simulink model "px4_controllers_IARTF"  (R2018a)
settings: Solver=ode4  StartTime=0.0  StopTime=sim_time  FixedStep=1/sim_freq  MaxStep=0.0025  MinStep=0.0005  RelTol=1e-3
values from neighbouring files (symbols this model uses):
  C_D = [0.025; 0.025; 0.025]    [quad_parameters_IARTF.m]    (also in quad_parameters_SLADe.m = [0.5; 0.5; 0.5])
  d = 0.1275    [quad_parameters_IARTF.m]    (also in quad_parameters_SLADe.m = 0.465)
  d_step_time = 0    [init_sim.m]
  d_step_val = 0    [init_sim.m]
  e_step_time = 0    [init_sim.m]
  e_step_val = 0    [init_sim.m]
  g = 9.80665    [init_sim.m]
  K_d_D = 0    [controller_gains_IARTF.m]
  K_d_I = 0    [controller_gains_IARTF.m]
  K_d_P = 1.5    [controller_gains_IARTF.m]
  K_e_D = 0    [controller_gains_IARTF.m]
  K_e_I = 0    [controller_gains_IARTF.m]
  K_e_P = 1.5    [controller_gains_IARTF.m]
  K_n_D = 0    [controller_gains_IARTF.m]
  K_n_I = 0    [controller_gains_IARTF.m]
  K_n_P = 1.5    [controller_gains_IARTF.m]
  K_p_D = 0.0135    [controller_gains_IARTF.m]
  K_p_I = 0.789    [controller_gains_IARTF.m]
  K_p_P = 1.466    [controller_gains_IARTF.m]
  K_phi_D = 0    [controller_gains_IARTF.m]
  K_phi_I = 0    [controller_gains_IARTF.m]
  K_phi_P = 8    [controller_gains_IARTF.m]
  K_psi_D = 0    [controller_gains_IARTF.m]
  K_psi_I = 0    [controller_gains_IARTF.m]
  K_psi_P = 4    [controller_gains_IARTF.m]
  K_q_D = 0.0135    [controller_gains_IARTF.m]
  K_q_I = 0.789    [controller_gains_IARTF.m]
  K_q_P = 1.466    [controller_gains_IARTF.m]
  K_r_D = 0    [controller_gains_IARTF.m]
  K_r_I = 0.564    [controller_gains_IARTF.m]
  K_r_P = 1.354    [controller_gains_IARTF.m]
  K_theta_D = 0    [controller_gains_IARTF.m]
  K_theta_I = 0    [controller_gains_IARTF.m]
  K_theta_P = 8    [controller_gains_IARTF.m]
  K_u_D = 0.1128    [controller_gains_IARTF.m]
  K_u_I = 0.2256    [controller_gains_IARTF.m]
  K_u_P = 1.6922    [controller_gains_IARTF.m]
  K_v_D = 0.1128    [controller_gains_IARTF.m]
  K_v_I = 0.2256    [controller_gains_IARTF.m]
  K_v_P = 1.6922    [controller_gains_IARTF.m]
  K_w_D = 0    [controller_gains_IARTF.m]
  K_w_I = 0.15    [controller_gains_IARTF.m]
  K_w_P = 0.8    [controller_gains_IARTF.m]
  m = 1.15    [quad_parameters_IARTF.m]    (also in quad_parameters_SLADe.m = 15)
  n_step_time = 0    [init_sim.m]
  n_step_val = 0    [init_sim.m]
  pitch_rate_step_time = 0    [init_sim.m]
  pitch_rate_step_val = 0    [init_sim.m]
  pitch_step_time = 0    [init_sim.m]
  pitch_step_val = 0    [init_sim.m]
  r_D = 0.115*0.375    (= 0.043125)    [quad_parameters_IARTF.m]    (also in quad_parameters_SLADe.m = 0.18)
  R_LD = 10    [init_sim.m]
  rho = 1.225    [init_sim.m]
  roll_rate_step_time = 0    [init_sim.m]
  roll_rate_step_val = 0    [init_sim.m]
  roll_step_time = 0    [init_sim.m]
  roll_step_val = 0    [init_sim.m]
  vx_step_time = 0    [init_sim.m]
  vx_step_val = 0    [init_sim.m]
  vy_step_time = 0    [init_sim.m]
  vy_step_val = 0    [init_sim.m]
  vz_step_time = 0    [init_sim.m]
  vz_step_val = 0    [init_sim.m]
  yaw_rate_step_time = 0    [init_sim.m]
  yaw_rate_step_val = 0    [init_sim.m]
  yaw_step_time = 0    [init_sim.m]
  yaw_step_val = 0    [init_sim.m]
undefined symbols (not defined in the file or in its folder): A_D, Eul_init, I_b, NED_init, PQR_init, tau, UVW_init
libraries: peGeneralControl x1
settings Model: Creator=Martin  LastModifiedBy=jjr

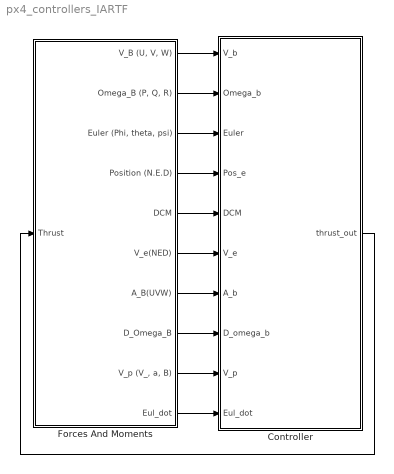
== system px4_controllers_IARTF ==
  Controller : Subsystem
  Forces And Moments : Subsystem
  wires:
  Forces And Moments/1("V_B (U, V, W)") -> Controller/1(V_b)
  Forces And Moments/2("Omega_B (P, Q, R)") -> Controller/2(Omega_b)
  Forces And Moments/3("Euler (Phi, theta, psi)") -> Controller/3(Euler)
  Forces And Moments/4(Position (N.E.D)) -> Controller/4(Pos_e)
  Forces And Moments/5(DCM) -> Controller/5(DCM)
  Forces And Moments/6(V_e(NED)) -> Controller/6(V_e)
  Forces And Moments/7(A_B(UVW)) -> Controller/7(A_b)
  Forces And Moments/8(D_Omega_B) -> Controller/8(D_omega_b)
  Forces And Moments/9("V_p (V_, a, B)") -> Controller/9(V_p)
  Forces And Moments/10(Eul_dot) -> Controller/10(Eul_dot)
  Controller/1(thrust_out) -> Forces And Moments/1(Thrust)

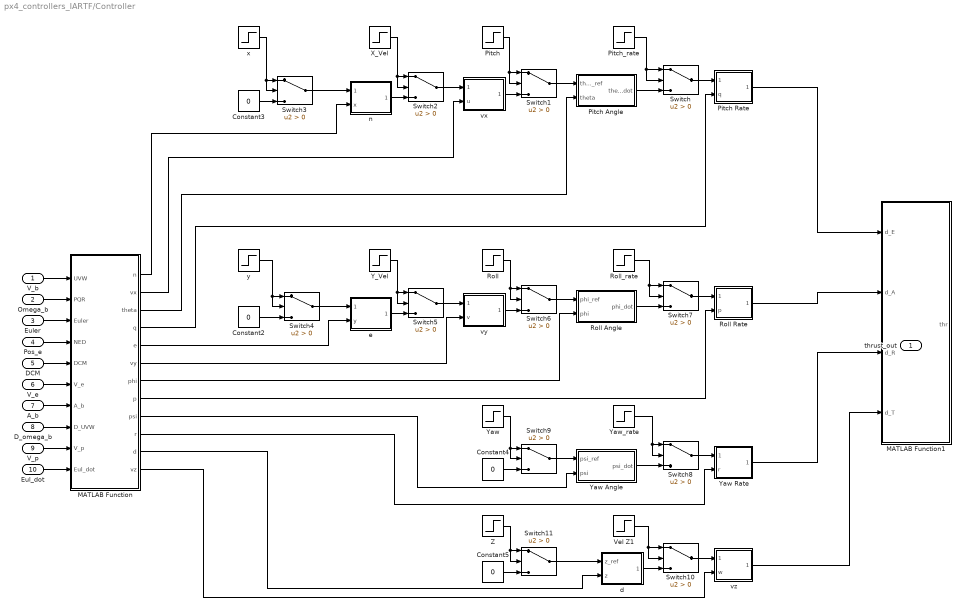
== system px4_controllers_IARTF/Controller ==
  V_b : Inport
  Omega_b : Inport  Port=2
  Euler : Inport  Port=3
  Pos_e : Inport  Port=4
  DCM : Inport  Port=5
  V_e : Inport  Port=6
  A_b : Inport  Port=7
  D_omega_b : Inport  Port=8
  V_p : Inport  Port=9
  Eul_dot : Inport  Port=10
  Constant{2..5} (4 alike) : Constant  Value=0
  MATLAB Function : MATLAB Function  TreatAsAtomicUnit=on
  MATLAB Function1 : MATLAB Function  TreatAsAtomicUnit=on
  Pitch : Step  Time=pitch_step_time  After=pitch_step_val  SampleTime=0
  Pitch Angle : Subsystem
  Pitch Rate : Subsystem
  Pitch_rate : Step  Time=pitch_rate_step_time  After=pitch_rate_step_val  SampleTime=0
  Roll : Step  Time=roll_step_time  After=roll_step_val  SampleTime=0
  Roll Angle : Subsystem
  Roll Rate : Subsystem
  Roll_rate : Step  Time=roll_rate_step_time  After=roll_rate_step_val  SampleTime=0
  Switch{,1..11} (12 alike) : Switch  Criteria=u2 > Threshold
  Vel Z1 : Step  Time=vz_step_time  After=vz_step_val  SampleTime=0
  X_Vel : Step  Time=vx_step_time  After=vx_step_val  SampleTime=0
  Y_Vel : Step  Time=vy_step_time  After=vy_step_val  SampleTime=0
  Yaw : Step  Time=yaw_step_time  After=yaw_step_val  SampleTime=0
  Yaw Angle : Subsystem
  Yaw Rate : Subsystem
  Yaw_rate : Step  Time=yaw_rate_step_time  After=yaw_rate_step_val  SampleTime=0
  Z : Step  Time=d_step_time  After=d_step_val  SampleTime=0
  d : Subsystem
  e : Subsystem
  n : Subsystem
  vx : Subsystem
  vy : Subsystem
  vz : Subsystem
  x : Step  Time=n_step_time  After=n_step_val  SampleTime=0
  y : Step  Time=e_step_time  After=e_step_val  SampleTime=0
  thrust_out : Outport
  wires:
  Switch2/1 -> vx/1(u_ref)
  Pitch/1 -> Switch1/2, Switch1/1
  Pitch_rate/1 -> Switch/2, Switch/1
  Pitch Angle/1(theta_dot) -> Switch/3
  vx/1(u_dot) -> Switch1/3
  d/1(d_dot) -> Switch10/3
  Switch11/1 -> d/1(z_ref)
  Yaw/1 -> Switch9/2, Switch9/1
  e/1(y_dot) -> Switch5/3
  Z/1 -> Switch11/2, Switch11/1
  Constant2/1 -> Switch4/3
  Yaw Angle/1(psi_dot) -> Switch8/3
  Switch3/1 -> n/1(X_ref)
  n/1(x_dot) -> Switch2/3
  Roll Rate/1(p_dot) -> MATLAB Function1/2(d_A)
  Yaw_rate/1 -> Switch8/2, Switch8/1
  X_Vel/1 -> Switch2/2, Switch2/1
  vy/1(v_dot) -> Switch6/3
  Switch4/1 -> e/1(Y_ref)
  Constant4/1 -> Switch9/3
  Vel Z1/1 -> Switch10/2, Switch10/1
  Pitch Rate/1(q_dot) -> MATLAB Function1/1(d_E)
  Constant3/1 -> Switch3/3
  Switch5/1 -> vy/1(v_ref)
  Switch9/1 -> Yaw Angle/1(psi_ref)
  Y_Vel/1 -> Switch5/1, Switch5/2
  y/1 -> Switch4/2, Switch4/1
  Switch6/1 -> Roll Angle/1(phi_ref)
  Switch7/1 -> Roll Rate/1(p_ref)
  Switch10/1 -> vz/1(w_ref)
  x/1 -> Switch3/2, Switch3/1
  Switch8/1 -> Yaw Rate/1(r_ref)
  Switch1/1 -> Pitch Angle/1(theta_ref)
  Roll Angle/1(phi_dot) -> Switch7/3
  Roll/1 -> Switch6/1, Switch6/2
  Roll_rate/1 -> Switch7/2, Switch7/1
  Constant5/1 -> Switch11/3
  Yaw Rate/1(r_dot) -> MATLAB Function1/3(d_R)
  Switch/1 -> Pitch Rate/1(q_ref)
  Eul_dot/1 -> MATLAB Function/10(Eul_dot)
  V_b/1 -> MATLAB Function/1(UVW)
  Omega_b/1 -> MATLAB Function/2(PQR)
  Euler/1 -> MATLAB Function/3(Euler)
  Pos_e/1 -> MATLAB Function/4(NED)
  DCM/1 -> MATLAB Function/5(DCM)
  V_e/1 -> MATLAB Function/6(V_e)
  A_b/1 -> MATLAB Function/7(A_b)
  D_omega_b/1 -> MATLAB Function/8(D_UVW)
  V_p/1 -> MATLAB Function/9(V_p)
  MATLAB Function/1(n) -> n/2(x)
  MATLAB Function/2(vx) -> vx/2(u)
  MATLAB Function/3(theta) -> Pitch Angle/2(theta)
  MATLAB Function/4(q) -> Pitch Rate/2(q)
  MATLAB Function/5(e) -> e/2(y)
  MATLAB Function/6(vy) -> vy/2(v)
  MATLAB Function/7(phi) -> Roll Angle/2(phi)
  MATLAB Function/8(p) -> Roll Rate/2(p)
  MATLAB Function/9(psi) -> Yaw Angle/2(psi)
  MATLAB Function/10(r) -> Yaw Rate/2(r)
  vz/1(w_dot) -> MATLAB Function1/4(d_T)
  MATLAB Function/11(d) -> d/2(z)
  MATLAB Function/12(vz) -> vz/2(w)

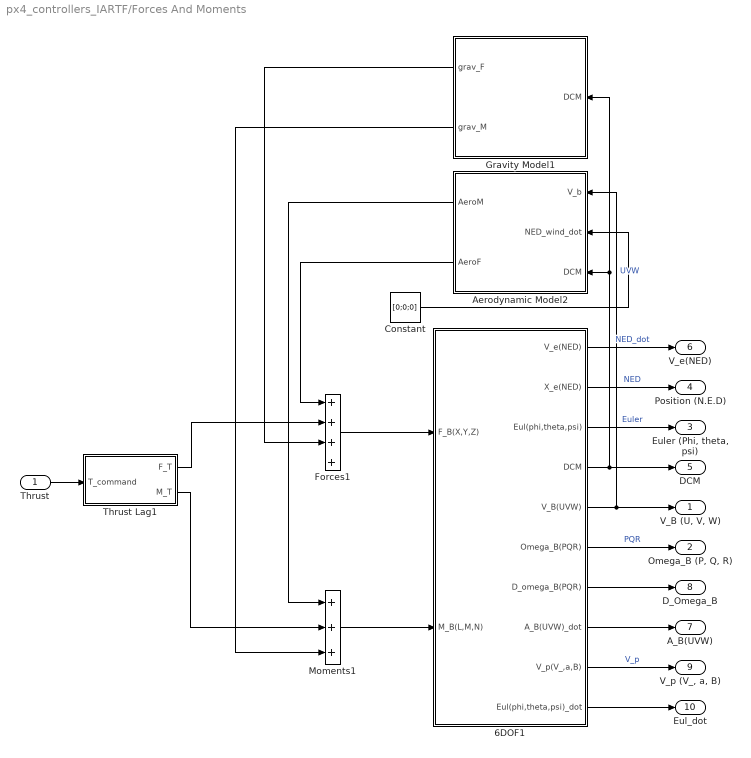
== system px4_controllers_IARTF/Forces And Moments ==
  Thrust : Inport
  6DOF1 : Subsystem
  Aerodynamic Model2 : MATLAB Function  TreatAsAtomicUnit=on
  Constant : Constant  Value=[0;0;0]
  Forces1 : Sum  Inputs=++++  RndMeth=Nearest
  Gravity Model1 : MATLAB Function  TreatAsAtomicUnit=on
  Moments1 : Sum  Inputs=+++  RndMeth=Nearest
  Thrust Lag1 : Subsystem
  "V_B (U, V, W)" : Outport
  "Omega_B (P, Q, R)" : Outport  Port=2
  "Euler (Phi, theta, psi)" : Outport  Port=3
  Position (N.E.D) : Outport  Port=4
  DCM : Outport  Port=5
  V_e(NED) : Outport  Port=6
  A_B(UVW) : Outport  Port=7
  D_Omega_B : Outport  Port=8
  "V_p (V_, a, B)" : Outport  Port=9
  Eul_dot : Outport  Port=10
  wires:
  Thrust/1 -> Thrust Lag1/1(T_command)
  6DOF1/3(Eul(phi,theta,psi)) -> "Euler (Phi, theta, psi)"/1  "Euler"
  Constant/1 -> Aerodynamic Model2/2(NED_wind_dot)
  Aerodynamic Model2/1(AeroM) -> Moments1/1
  Moments1/1 -> 6DOF1/2(M_B(L,M,N))
  Thrust Lag1/1(F_T) -> Forces1/2
  Gravity Model1/2(grav_M) -> Moments1/3
  Thrust Lag1/2(M_T) -> Moments1/2
  6DOF1/4(DCM) -> Gravity Model1/1(DCM), Aerodynamic Model2/3(DCM), DCM/1
  6DOF1/9(V_p(V_,a,B)) -> "V_p (V_, a, B)"/1  "V_p"
  Forces1/1 -> 6DOF1/1(F_B(X,Y,Z))
  Aerodynamic Model2/2(AeroF) -> Forces1/1
  6DOF1/6(Omega_B(PQR)) -> "Omega_B (P, Q, R)"/1  "PQR"
  6DOF1/10(Eul(phi,theta,psi)_dot) -> Eul_dot/1
  6DOF1/8(A_B(UVW)_dot) -> A_B(UVW)/1
  Gravity Model1/1(grav_F) -> Forces1/3
  6DOF1/5(V_B(UVW)) -> "V_B (U, V, W)"/1, Aerodynamic Model2/1(V_b)  "UVW"
  6DOF1/2(X_e(NED)) -> Position (N.E.D)/1  "NED"
  6DOF1/7(D_omega_B(PQR)) -> D_Omega_B/1
  6DOF1/1(V_e(NED)) -> V_e(NED)/1  "NED_dot"

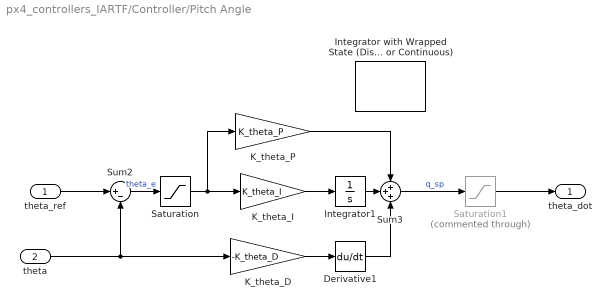
== system px4_controllers_IARTF/Controller/Pitch Angle ==
  theta_ref : Inport
  theta : Inport  Port=2
  Derivative1 : Derivative
  Integrator with Wrapped State (Discrete or Continuous) : peGeneralControl/Integrator with Wrapped State (Discrete or Continuous)  OverrideUsingVariant=Discrete  WrappedStateUpperValue=2*pi  WrappedStateLowerValue=0  x0=0  Ts=-1
  Integrator1 : Integrator
  K_theta_D : Gain  Gain=-K_theta_D
  K_theta_I : Gain  Gain=K_theta_I
  K_theta_P : Gain  Gain=K_theta_P
  Saturation : Saturate  UpperLimit=pi/6  LowerLimit=-pi/6
  Saturation1 : Saturate  Commented=through  UpperLimit=1  LowerLimit=-1
  Sum2 : Sum  Inputs=|+-
  Sum3 : Sum  Inputs=+++
  theta_dot : Outport
  wires:
  Saturation1/1 -> theta_dot/1
  Saturation/1 -> K_theta_P/1, K_theta_I/1
  Derivative1/1 -> Sum3/3
  Integrator1/1 -> Sum3/2
  Sum3/1 -> Saturation1/1  "q_sp"
  K_theta_I/1 -> Integrator1/1
  Sum2/1 -> Saturation/1  "theta_e"
  K_theta_P/1 -> Sum3/1
  K_theta_D/1 -> Derivative1/1
  theta_ref/1 -> Sum2/1
  theta/1 -> K_theta_D/1, Sum2/2

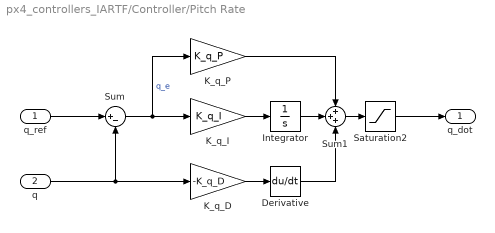
== system px4_controllers_IARTF/Controller/Pitch Rate ==
  q_ref : Inport
  q : Inport  Port=2
  Derivative : Derivative
  Integrator : Integrator
  K_q_D : Gain  Gain=-K_q_D
  K_q_I : Gain  Gain=K_q_I
  "K_q_P " : Gain  Gain=K_q_P
  Saturation2 : Saturate  UpperLimit=1  LowerLimit=-1
  Sum : Sum  Inputs=|+-
  Sum1 : Sum  Inputs=+++
  q_dot : Outport
  wires:
  Integrator/1 -> Sum1/2
  Derivative/1 -> Sum1/3
  "K_q_P "/1 -> Sum1/1
  K_q_D/1 -> Derivative/1
  K_q_I/1 -> Integrator/1
  Sum1/1 -> Saturation2/1
  Sum/1 -> "K_q_P "/1, K_q_I/1  "q_e"
  q_ref/1 -> Sum/1
  Saturation2/1 -> q_dot/1
  q/1 -> K_q_D/1, Sum/2

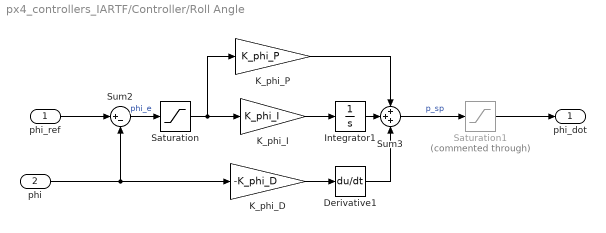
== system px4_controllers_IARTF/Controller/Roll Angle ==
  phi_ref : Inport
  phi : Inport  Port=2
  Derivative1 : Derivative
  Integrator1 : Integrator
  K_phi_D : Gain  Gain=-K_phi_D
  K_phi_I : Gain  Gain=K_phi_I
  K_phi_P : Gain  Gain=K_phi_P
  Saturation : Saturate  UpperLimit=pi/6  LowerLimit=-pi/6
  Saturation1 : Saturate  Commented=through  UpperLimit=1  LowerLimit=-1
  Sum2 : Sum  Inputs=|+-
  Sum3 : Sum  Inputs=+++
  phi_dot : Outport
  wires:
  Saturation1/1 -> phi_dot/1
  Saturation/1 -> K_phi_P/1, K_phi_I/1
  Derivative1/1 -> Sum3/3
  Integrator1/1 -> Sum3/2
  Sum3/1 -> Saturation1/1  "p_sp"
  K_phi_I/1 -> Integrator1/1
  Sum2/1 -> Saturation/1  "phi_e"
  K_phi_P/1 -> Sum3/1
  K_phi_D/1 -> Derivative1/1
  phi_ref/1 -> Sum2/1
  phi/1 -> K_phi_D/1, Sum2/2

== system px4_controllers_IARTF/Controller/Roll Rate ==
  p_ref : Inport
  p : Inport  Port=2
  Derivative : Derivative
  Integrator : Integrator
  K_p_D : Gain  Gain=-K_p_D
  K_p_I : Gain  Gain=K_p_I
  "K_p_P " : Gain  Gain=K_p_P
  Saturation2 : Saturate  UpperLimit=1  LowerLimit=-1
  Sum : Sum  Inputs=|+-
  Sum1 : Sum  Inputs=+++
  p_dot : Outport
  wires:
  Integrator/1 -> Sum1/2
  Derivative/1 -> Sum1/3
  "K_p_P "/1 -> Sum1/1
  K_p_D/1 -> Derivative/1
  K_p_I/1 -> Integrator/1
  Sum1/1 -> Saturation2/1
  Sum/1 -> "K_p_P "/1, K_p_I/1  "p_e"
  p_ref/1 -> Sum/1
  Saturation2/1 -> p_dot/1
  p/1 -> K_p_D/1, Sum/2

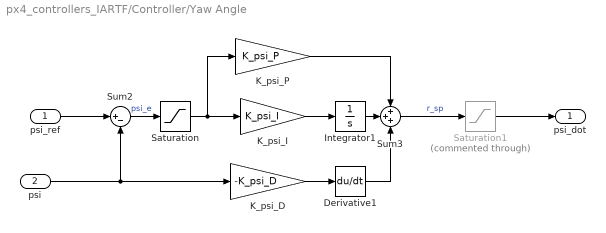
== system px4_controllers_IARTF/Controller/Yaw Angle ==
  psi_ref : Inport
  psi : Inport  Port=2
  Derivative1 : Derivative
  Integrator1 : Integrator
  K_psi_D : Gain  Gain=-K_psi_D
  K_psi_I : Gain  Gain=K_psi_I
  K_psi_P : Gain  Gain=K_psi_P
  Saturation : Saturate  UpperLimit=pi/6  LowerLimit=-pi/6
  Saturation1 : Saturate  Commented=through  UpperLimit=1  LowerLimit=-1
  Sum2 : Sum  Inputs=|+-
  Sum3 : Sum  Inputs=+++
  psi_dot : Outport
  wires:
  Saturation1/1 -> psi_dot/1
  Saturation/1 -> K_psi_P/1, K_psi_I/1
  Derivative1/1 -> Sum3/3
  Integrator1/1 -> Sum3/2
  Sum3/1 -> Saturation1/1  "r_sp"
  K_psi_I/1 -> Integrator1/1
  Sum2/1 -> Saturation/1  "psi_e"
  K_psi_P/1 -> Sum3/1
  K_psi_D/1 -> Derivative1/1
  psi_ref/1 -> Sum2/1
  psi/1 -> K_psi_D/1, Sum2/2

== system px4_controllers_IARTF/Controller/Yaw Rate ==
  r_ref : Inport
  r : Inport  Port=2
  Derivative : Derivative
  Integrator : Integrator
  K_r_D : Gain  Gain=-K_r_D
  K_r_I : Gain  Gain=K_r_I
  "K_r_P " : Gain  Gain=K_r_P
  Saturation2 : Saturate  UpperLimit=1  LowerLimit=-1
  Sum : Sum  Inputs=|+-
  Sum1 : Sum  Inputs=+++
  r_dot : Outport
  wires:
  Integrator/1 -> Sum1/2
  Derivative/1 -> Sum1/3
  "K_r_P "/1 -> Sum1/1
  K_r_D/1 -> Derivative/1
  K_r_I/1 -> Integrator/1
  Sum1/1 -> Saturation2/1
  Sum/1 -> "K_r_P "/1, K_r_I/1  "r_e"
  r_ref/1 -> Sum/1
  Saturation2/1 -> r_dot/1
  r/1 -> K_r_D/1, Sum/2

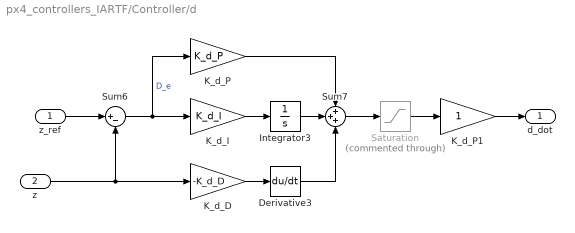
== system px4_controllers_IARTF/Controller/d ==
  z_ref : Inport
  z : Inport  Port=2
  Derivative3 : Derivative
  Integrator3 : Integrator
  K_d_D : Gain  Gain=-K_d_D
  K_d_I : Gain  Gain=K_d_I
  K_d_P : Gain  Gain=K_d_P
  K_d_P1 : Gain
  Saturation : Saturate  Commented=through  UpperLimit=5  LowerLimit=-5
  Sum6 : Sum  Inputs=|+-
  Sum7 : Sum  Inputs=+++
  d_dot : Outport
  wires:
  Saturation/1 -> K_d_P1/1
  K_d_I/1 -> Integrator3/1
  Derivative3/1 -> Sum7/3
  K_d_D/1 -> Derivative3/1
  K_d_P/1 -> Sum7/1
  Integrator3/1 -> Sum7/2
  Sum6/1 -> K_d_P/1, K_d_I/1  "D_e"
  Sum7/1 -> Saturation/1
  z_ref/1 -> Sum6/1
  z/1 -> Sum6/2, K_d_D/1
  K_d_P1/1 -> d_dot/1

== system px4_controllers_IARTF/Controller/e ==
  Y_ref : Inport
  y : Inport  Port=2
  Derivative3 : Derivative
  Integrator3 : Integrator
  K_e_D : Gain  Gain=-K_e_D
  K_e_I : Gain  Gain=K_e_I
  K_e_P : Gain  Gain=K_e_P
  Saturation : Saturate  Commented=through  UpperLimit=5  LowerLimit=-5
  Sum6 : Sum  Inputs=|+-
  Sum7 : Sum  Inputs=+++
  y_dot : Outport
  wires:
  Saturation/1 -> y_dot/1
  K_e_I/1 -> Integrator3/1
  Derivative3/1 -> Sum7/3
  K_e_D/1 -> Derivative3/1
  K_e_P/1 -> Sum7/1
  Integrator3/1 -> Sum7/2
  Sum6/1 -> K_e_P/1, K_e_I/1  "E_e"
  Sum7/1 -> Saturation/1
  Y_ref/1 -> Sum6/1
  y/1 -> K_e_D/1, Sum6/2

== system px4_controllers_IARTF/Controller/n ==
  X_ref : Inport
  x : Inport  Port=2
  Derivative3 : Derivative
  Integrator3 : Integrator
  K_n_D : Gain  Gain=-K_n_D
  K_n_I : Gain  Gain=K_n_I
  K_n_P : Gain  Gain=K_n_P
  Saturation : Saturate  Commented=through  UpperLimit=5  LowerLimit=-5
  Sum6 : Sum  Inputs=|+-
  Sum7 : Sum  Inputs=+++
  x_dot : Outport
  wires:
  Saturation/1 -> x_dot/1
  K_n_I/1 -> Integrator3/1
  Derivative3/1 -> Sum7/3
  K_n_D/1 -> Derivative3/1
  K_n_P/1 -> Sum7/1
  Integrator3/1 -> Sum7/2
  Sum6/1 -> K_n_P/1, K_n_I/1  "N_e"
  Sum7/1 -> Saturation/1
  X_ref/1 -> Sum6/1
  x/1 -> K_n_D/1, Sum6/2

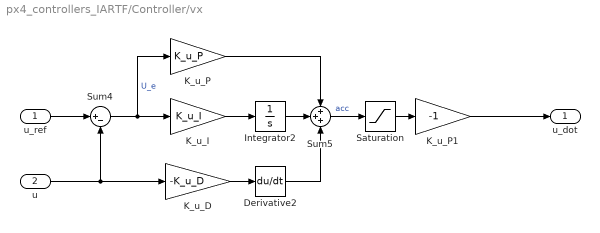
== system px4_controllers_IARTF/Controller/vx ==
  u_ref : Inport
  u : Inport  Port=2
  Derivative2 : Derivative
  Integrator2 : Integrator
  K_u_D : Gain  Gain=-K_u_D
  K_u_I : Gain  Gain=K_u_I
  K_u_P : Gain  Gain=K_u_P
  K_u_P1 : Gain  Gain=-1
  Saturation : Saturate  UpperLimit=5  LowerLimit=-5
  Sum4 : Sum  Inputs=|+-
  Sum5 : Sum  Inputs=+++
  u_dot : Outport
  wires:
  K_u_I/1 -> Integrator2/1
  K_u_P/1 -> Sum5/1
  K_u_D/1 -> Derivative2/1
  Sum4/1 -> K_u_P/1, K_u_I/1  "U_e"
  Sum5/1 -> Saturation/1  "acc"
  Derivative2/1 -> Sum5/3
  Integrator2/1 -> Sum5/2
  u/1 -> K_u_D/1, Sum4/2
  u_ref/1 -> Sum4/1
  Saturation/1 -> K_u_P1/1
  K_u_P1/1 -> u_dot/1

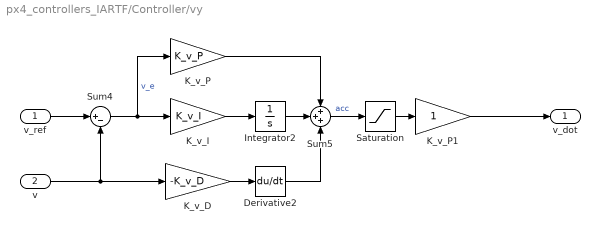
== system px4_controllers_IARTF/Controller/vy ==
  v_ref : Inport
  v : Inport  Port=2
  Derivative2 : Derivative
  Integrator2 : Integrator
  K_v_D : Gain  Gain=-K_v_D
  K_v_I : Gain  Gain=K_v_I
  K_v_P : Gain  Gain=K_v_P
  K_v_P1 : Gain
  Saturation : Saturate  UpperLimit=5  LowerLimit=-5
  Sum4 : Sum  Inputs=|+-
  Sum5 : Sum  Inputs=+++
  v_dot : Outport
  wires:
  K_v_I/1 -> Integrator2/1
  K_v_P/1 -> Sum5/1
  K_v_D/1 -> Derivative2/1
  Sum4/1 -> K_v_P/1, K_v_I/1  "v_e"
  Sum5/1 -> Saturation/1  "acc"
  Derivative2/1 -> Sum5/3
  Integrator2/1 -> Sum5/2
  v/1 -> K_v_D/1, Sum4/2
  v_ref/1 -> Sum4/1
  Saturation/1 -> K_v_P1/1
  K_v_P1/1 -> v_dot/1

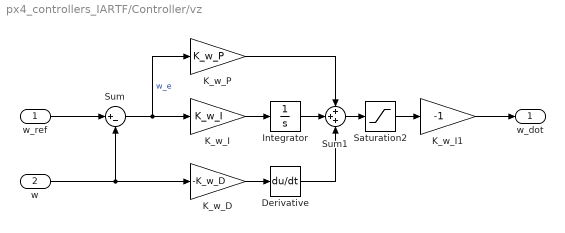
== system px4_controllers_IARTF/Controller/vz ==
  w_ref : Inport
  w : Inport  Port=2
  Derivative : Derivative
  Integrator : Integrator
  K_w_D : Gain  Gain=-K_w_D
  K_w_I : Gain  Gain=K_w_I
  K_w_I1 : Gain  Gain=-1
  "K_w_P " : Gain  Gain=K_w_P
  Saturation2 : Saturate  UpperLimit=1  LowerLimit=-1
  Sum : Sum  Inputs=|+-
  Sum1 : Sum  Inputs=+++
  w_dot : Outport
  wires:
  Integrator/1 -> Sum1/2
  Derivative/1 -> Sum1/3
  "K_w_P "/1 -> Sum1/1
  K_w_D/1 -> Derivative/1
  K_w_I/1 -> Integrator/1
  Sum1/1 -> Saturation2/1
  Sum/1 -> "K_w_P "/1, K_w_I/1  "w_e"
  w_ref/1 -> Sum/1
  Saturation2/1 -> K_w_I1/1
  w/1 -> K_w_D/1, Sum/2
  K_w_I1/1 -> w_dot/1

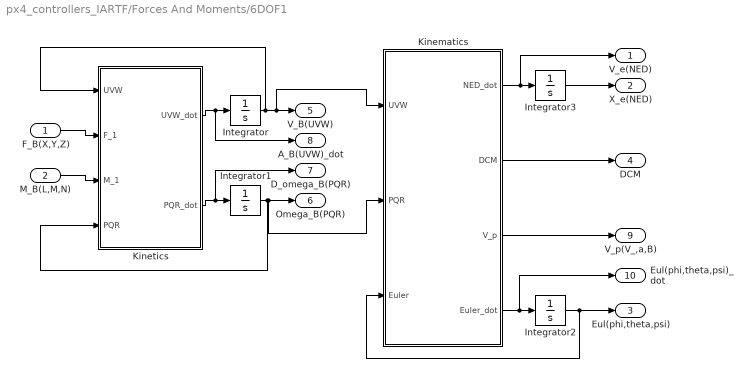
== system px4_controllers_IARTF/Forces And Moments/6DOF1 ==
  F_B(X,Y,Z) : Inport
  M_B(L,M,N) : Inport  Port=2
  Integrator : Integrator  InitialCondition=UVW_init
  Integrator1 : Integrator  InitialCondition=PQR_init
  Integrator2 : Integrator  InitialCondition=Eul_init  WrapState=on  WrappedStateUpperValue=pi.*[1;1;1]  WrappedStateLowerValue=-pi.*[1;1;1]
  Integrator3 : Integrator  InitialCondition=NED_init
  Kinematics : MATLAB Function  TreatAsAtomicUnit=on
  Kinetics : MATLAB Function  TreatAsAtomicUnit=on
  V_e(NED) : Outport
  X_e(NED) : Outport  Port=2
  Eul(phi,theta,psi) : Outport  Port=3
  DCM : Outport  Port=4
  V_B(UVW) : Outport  Port=5
  Omega_B(PQR) : Outport  Port=6
  D_omega_B(PQR) : Outport  Port=7
  A_B(UVW)_dot : Outport  Port=8
  V_p(V_,a,B) : Outport  Port=9
  Eul(phi,theta,psi)_dot : Outport  Port=10
  wires:
  Kinetics/1(UVW_dot) -> A_B(UVW)_dot/1, Integrator/1
  Kinetics/2(PQR_dot) -> D_omega_B(PQR)/1, Integrator1/1
  Integrator1/1 -> Kinetics/4(PQR), Omega_B(PQR)/1, Kinematics/2(PQR)
  Integrator/1 -> Kinetics/1(UVW), Kinematics/1(UVW), V_B(UVW)/1
  M_B(L,M,N)/1 -> Kinetics/3(M_1)
  F_B(X,Y,Z)/1 -> Kinetics/2(F_1)
  Kinematics/4(Euler_dot) -> Eul(phi,theta,psi)_dot/1, Integrator2/1
  Kinematics/3(V_p) -> V_p(V_,a,B)/1
  Kinematics/2(DCM) -> DCM/1
  Kinematics/1(NED_dot) -> V_e(NED)/1, Integrator3/1
  Integrator3/1 -> X_e(NED)/1
  Integrator2/1 -> Kinematics/3(Euler), Eul(phi,theta,psi)/1

== system px4_controllers_IARTF/Forces And Moments/Thrust Lag1 ==
  T_command : Inport
  Integrator : Integrator  InitialCondition=[1;1;1;1].*0
  Trust Model : MATLAB Function  TreatAsAtomicUnit=on
  F_T : Outport
  M_T : Outport  Port=2
  wires:
  T_command/1 -> Trust Model/2(Thrust_command)
  Trust Model/3(Thrust_M) -> M_T/1
  Trust Model/2(Thrust_F) -> F_T/1
  Trust Model/1(T_dot) -> Integrator/1
  Integrator/1 -> Trust Model/1(Thrust_mag)

== matlab function px4_controllers_IARTF/Controller/MATLAB Function1 ==
  data: d_E input; d_A input; d_R input; d_T input; thr output; g parameter; m parameter
function thr = fcn(d_E, d_A, d_R, d_T , g, m)
motor_max = 0.5*m*g;
comand = [d_T; d_A; d_E; d_R];
thr = virtual_controls_mat*comand;
thr = motor_max.*thr;

== matlab function px4_controllers_IARTF/Controller/MATLAB Function ==
  data: UVW input; n output; PQR input; Euler input; NED input; DCM input; V_e input; A_b input; D_UVW input; V_p input; Eul_dot input; vx output; theta output; q output; e output; vy output; phi output; p output; psi output; r output; d output; vz output
function [n,vx,theta,q,e,vy,phi,p,psi,r,d,vz] = fcn(UVW,PQR,Euler,NED,DCM,V_e,A_b,D_UVW,V_p,Eul_dot)

n = NED(1);
vx = UVW(1);
theta = Euler(2);
q = PQR(2);
e = NED(2);
vy = UVW(2);
phi = Euler(1);
p = PQR(1);
psi = Euler(3);
r = PQR(3);
d = NED(3);
vz = UVW(3);

== matlab function px4_controllers_IARTF/Forces And Moments/6DOF1/Kinematics ==
  settings: updateMethod=CONTINUOUS
  data: UVW input; NED_dot output; PQR input; Euler input; DCM output; V_p output; Euler_dot output
function [NED_dot, DCM, V_p, Euler_dot]  = fcn(UVW, PQR, Euler)


U   = UVW(1);
V   = UVW(2);
W   = UVW(3);
P   = PQR(1);
Q   = PQR(2);
R   = PQR(3);
phi   = Euler(1);
theta = Euler(2);
psi   = Euler(3);

DCM  = [ cos(psi)*cos(theta),                                sin(psi)*cos(theta),                               -sin(theta); 
         cos(psi)*sin(theta)*sin(phi)-sin(psi)*cos(phi),     sin(psi)*sin(theta)*sin(phi)+cos(psi)*cos(phi),    cos(theta)*sin(phi);
         cos(psi)*sin(theta)*cos(phi)+sin(psi)*sin(phi),     sin(psi)*sin(theta)*cos(phi)-cos(psi)*sin(phi),  cos(theta)*cos(phi)];

NED_dot      = DCM'*[U;V;W];

temp = [ 1,     sin(phi)*tan(theta),    cos(phi)*tan(theta);
         0,     cos(phi),               -sin(phi); 
         0,     sin(phi)*sec(theta),    cos(phi)*sec(theta)];

Euler_dot = Euler;
temp         = temp*[P;Q;R];

Euler_dot(1) = temp(1);
Euler_dot(2) = temp(2);
Euler_dot(3) = temp(3);
V_p = zeros(3,1);
V_p(1) = sqrt(U.^2 + V.^2 + W.^2);
V_p(2) = atan2(W,U);
V_p(3) = asin(V/V_p(1));

== matlab function px4_controllers_IARTF/Forces And Moments/6DOF1/Kinetics ==
  settings: updateMethod=CONTINUOUS
  data: UVW input; UVW_dot output; F_1 input; M_1 input; PQR input; PQR_dot output; m parameter size=1; I_b parameter size=3
function [UVW_dot, PQR_dot]  = fcn(UVW, F_1,M_1, PQR, m, I_b)

Ixx = I_b(1);
Iyy = I_b(2);
Izz = I_b(3);
X   = F_1(1);
Y   = F_1(2);
Z   = F_1(3);
L   = M_1(1);
M   = M_1(2);
N   = M_1(3);
U   = UVW(1);
V   = UVW(2);
W   = UVW(3);
P   = PQR(1);
Q   = PQR(2);
R   = PQR(3);

UVW_dot      = zeros(3,1);
PQR_dot      = zeros(3,1);

UVW_dot(1,1) = (X/m) + (V*R) - (W*Q);
UVW_dot(2,1) = (Y/m) - (U*R) + (W*P);
UVW_dot(3,1) = (Z/m) + (U*Q) - (V*P);
PQR_dot(1,1) = (L - Q*R*(Izz-Iyy))/Ixx;
PQR_dot(2,1) = (M - P*R*(Ixx-Izz))/Iyy;
PQR_dot(3,1) = (N - P*Q*(Iyy-Ixx))/Izz;

== matlab function px4_controllers_IARTF/Forces And Moments/Aerodynamic Model2 ==
  settings: updateMethod=CONTINUOUS
  data: AeroM output; V_b input; NED_wind_dot input; DCM input; AeroF output; rho parameter; A_D parameter; C_D parameter
function [AeroM, AeroF] = fcn(V_b, NED_wind_dot, DCM, rho, A_D, C_D)

NED_wind_dot = DCM * NED_wind_dot;

F_d   = (0.5*rho).*A_D.*C_D;

UVW   = V_b - NED_wind_dot;

Force = F_d.*UVW.*abs(UVW);

AeroF       = [0;0;0];
AeroF(1)    =  -Force(1);
AeroF(2)    =  -Force(2);
AeroF(3)    =  -Force(3);

AeroM       = [0;0;0];

== matlab function px4_controllers_IARTF/Forces And Moments/Gravity Model1 ==
  settings: updateMethod=CONTINUOUS
  data: grav_F output; grav_M output; DCM input; m parameter; g parameter
function [grav_F, grav_M] = fcn(DCM, m, g)


grav_M = [0;0;0];

grav_F = DCM*[0;0;m*g];

== matlab function px4_controllers_IARTF/Forces And Moments/Thrust Lag1/Trust Model ==
  settings: updateMethod=CONTINUOUS
  data: Thrust_mag input; T_dot output; Thrust_command input; Thrust_F output; Thrust_M output; d parameter; R_LD parameter; r_D parameter; tau parameter
function [T_dot, Thrust_F, Thrust_M] = fcn( Thrust_mag,Thrust_command, d, R_LD, r_D, tau)

% T1_c = Thrust_command(1);
% T2_c = Thrust_command(2);
% T3_c = Thrust_command(3);
% T4_c = Thrust_command(4);
% 
% T1_m = Thrust_mag(1);
% T2_m = Thrust_mag(2);
% T3_m = Thrust_mag(3);
% T4_m = Thrust_mag(4);

T_dot = (Thrust_command-Thrust_mag)./tau;


T1 = Thrust_mag(1);
T2 = Thrust_mag(2);
T3 = Thrust_mag(3);
T4 = Thrust_mag(4);

Thrust_F = [0;0;0];
Thrust_M = [0;0;0];

Thrust_F(3) = -(T1 + T2 + T3 + T4);

% Thrust_M(1) = d * (-T1 + T2);
% Thrust_M(2) = d * (T3 - T4);
Thrust_M(1) = d * (-T1 + T2 + T3 - T4);
Thrust_M(2) = d * (T1 - T2 + T3 - T4);

Thrust_M(3) = r_D *(T1 + T2 - T3 - T4) /R_LD;
